simulink model "Three_Phase_Diode_Rectifier"  (R2024b)
settings: Solver=VariableStepAuto  StartTime=0.0  StopTime=1  RelTol=1e-3
libraries: spsDiodeLib x6, spsACVoltageSourceLib x3, spsSeriesRLCBranchLib x2, spsMeanLib x2, spsMultimeterLib x2, spsGroundLib x1, sps_lib x1
settings Model: Creator=User  LastModifiedBy=User

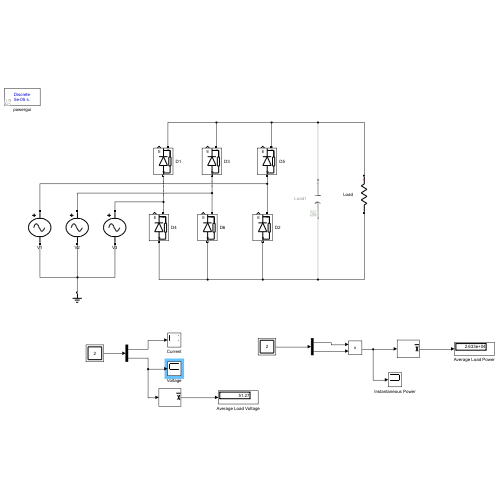
[thumbnail: Simulink's stored preview of the top-level diagram]
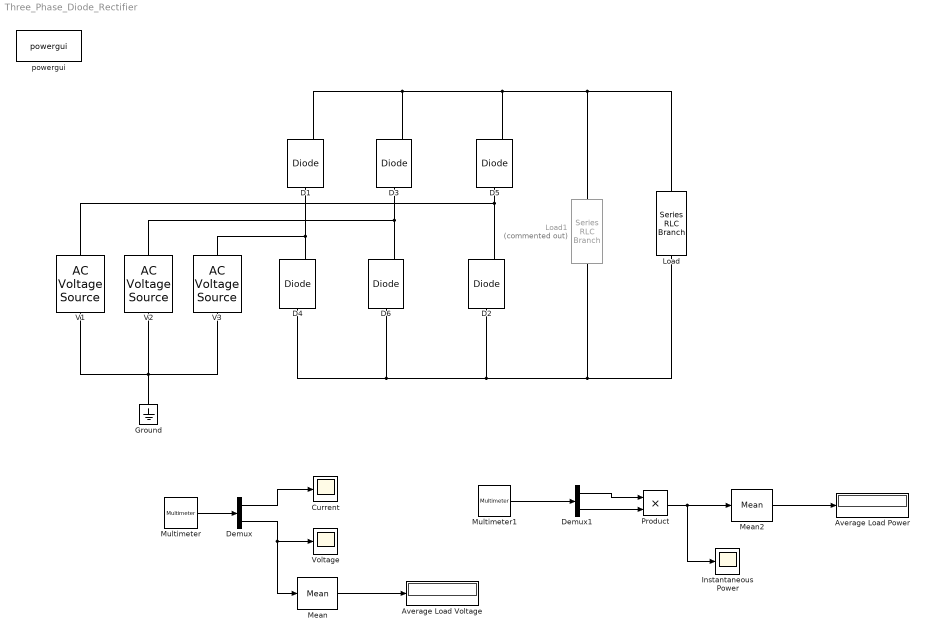
== system Three_Phase_Diode_Rectifier ==
  Average Load Power : Display
  Average Load Voltage : Display
  Current : Scope
  D{1..6} (6 alike) : spsDiodeLib/Diode  Ron=0.001  Lon=0  Vf=0.8  IC=0  UseSnubber=0  Rs=500  Cs=250e-9  Measurements=on
  Demux : Demux  Outputs=2
  Demux1 : Demux  Outputs=2
  Ground : spsGroundLib/Ground  LConnTagsString=a
  Instantaneous Power : Scope
  Load : spsSeriesRLCBranchLib/Series RLC Branch  LConnTagsString=__new0  RConnTagsString=__new0  BranchType=R  Resistance=10  Inductance=1e-3  SetiL0=off  InitialCurrent=0  Capacitance=1e-6  Setx0=off  InitialVoltage=0  Measurements=Branch voltage and current
  Load1 : spsSeriesRLCBranchLib/Series RLC Branch  Commented=on  LConnTagsString=__new0  RConnTagsString=__new0  BranchType=C  Resistance=10  Inductance=1e-3  SetiL0=off  InitialCurrent=0  Capacitance=30e-3  Setx0=off  InitialVoltage=0  Measurements=Branch voltage and current
  Mean : spsMeanLib/Mean  Freq=60  Vinit=0  Ts=0
  Mean2 : spsMeanLib/Mean  Freq=60  Vinit=0  Ts=0
  Multimeter : spsMultimeterLib/Multimeter  L=2  sel=[1 2]  yselected={}  Gain=[1 1]  OutputType=Complex  PlotAtSimulationStop=off  PhasorSimulation=off
  Multimeter1 : spsMultimeterLib/Multimeter  L=2  sel=[1 2]  yselected={}  Gain=[1 1]  OutputType=Complex  PlotAtSimulationStop=off  PhasorSimulation=off
  Product : Product
  V1 : spsACVoltageSourceLib/AC Voltage Source  Amplitude=311  Phase=0  Frequency=50  SampleTime=0  Measurements=None  BusType=swing  Pref=10e3  Qref=0  Qmin=-inf  Qmax=+inf
  V2 : spsACVoltageSourceLib/AC Voltage Source  Amplitude=311  Phase=-120  Frequency=50  SampleTime=0  Measurements=None  BusType=swing  Pref=10e3  Qref=0  Qmin=-inf  Qmax=+inf
  V3 : spsACVoltageSourceLib/AC Voltage Source  Amplitude=311  Phase=+120  Frequency=50  SampleTime=0  Measurements=None  BusType=swing  Pref=10e3  Qref=0  Qmin=-inf  Qmax=+inf
  Voltage : Scope
  powergui : sps_lib/powergui  Priority=1  SimulationMode=Discrete  SampleTime=50e-06  frequency=60  Iterations=50  frequencyindice=50  Pbase=100e6  ErrMax=1e-4  UnitsV=kV  UnitsW=MW  buscounter=0  FunctionMessages=off  echomessages=off  EnableUseOfTLC=off  CurrentSourceSwitches=off  DisableSnubberDevices=off  DisableRonSwitches=off  DisableVfSwitches=off  DisplayEquations=off  AutomaticDiscreteSolvers=off  SolverType=Tustin/Backward Euler (TBE)  Interpol=off  ExternalGateDelay=off  methode=off  Ts=100  x0status=blocks  SPID=on  SwTol=0  HookPort=off  NonlinearTolerance=1e-4  nMaxIteration=100  ContinueOnMaxIteration=off  RestoreLinks=warning  ResistiveCurrentMeasurement=off  Frange=[0:2:500]  Ylog=off  Xlog=on  ShowGrid=off  save=off  variable=ZData  structure=0  ZoomFFT=off  StartTime=0.0  cycles=1  DisplayStyle=1  fundamental=60  FreqAxis=off  MaxFrequency=1000  frequencyindicesteady=1  RmsSteady=1  display=off
  wires:
  Demux/1 -> Current/1
  Demux/2 -> Mean/1, Voltage/1
  Mean/1 -> Average Load Voltage/1
  Demux1/1 -> Product/1
  Demux1/2 -> Product/2
  Product/1 -> Instantaneous Power/1, Mean2/1
  Mean2/1 -> Average Load Power/1
  Multimeter/1 -> Demux/1
  Multimeter1/1 -> Demux1/1
  connections:
  V3/LConn1 -- Ground/LConn1 -- V2/LConn1 -- V1/LConn1
  D4/RConn1 -- V3/RConn1 -- D1/LConn1
  D6/RConn1 -- V2/RConn1 -- D3/LConn1
  D2/RConn1 -- V1/RConn1 -- D5/LConn1
  Load/RConn1 -- Load1/RConn1 -- D2/LConn1 -- D6/LConn1 -- D4/LConn1
  Load/LConn1 -- Load1/LConn1 -- D5/RConn1 -- D3/RConn1 -- D1/RConn1
